simulink model "TrajectoryFollowVehicleWith14DoF_"  (R2024b)
settings: Solver=VariableStepAuto  StartTime=0  StopTime=14  FixedStep=timeStep  RelTol=1e-3
PreLoadFcn:
  | useDynamicsStanley = false; %Simulink model to move according to the scenario trajectory.
  | vehicleVariant = "3DOF";
PostLoadFcn:
  | load(fullfile(matlabroot,'toolbox','driving','drivingdata','rrScenarioSimTypes.mat'));
  | helperSLTrajectoryFollowerWithRRScenarioSetup();
  | hegihtMap = "flat";
  | if isfile("pathFollowingUtil/gridMap_groundHeight_RT.mat")
  |     load("gridMap_groundHeight_RT.mat");
  | end
  | % if exist("z_2DTable", "var") && exist("xBreakPts", "var") && exist("yBreakPts", "var")
  | %     hegihtMap = "2DMap";
  | % end
  | % if isfile("CRG/crgRoad.crg")
  | %     crgData = crg_read('CRG/crgRoad.crg');
  | % end
InitFcn:
  | if ~exist("slBus42", "var")
  |     load("Bus_VehFdbk.mat");
  | end
StartFcn:
  | % set_param(bdroot, 'Profile', 'on');
StopFcn:
  | % set_param(bdroot, 'Profile', 'off');
  | % slprofreport(bdroot, 'report14DoF.html');
undefined symbols (not defined in the file or in its folder): control_timeStep, Defined, Ego, egoInitialPose, egoInitialPoseCG, egoInitialPoseRear, InitVehicle, Lane, lr, m, magnitude, max_dc, n, Pose, RRtimeStep, SceneData, steerGear, tau, tau2, timeStep, User, VehicleData, Velocity, X, xBreakPts, Y, yBreakPts, Z, z_2DTable
libraries: sm_lib x40, nesl_utility x25, simulink_extras x12, sm_vehicle_utilities_lib x7, roadrunnerscenario x6, drivingvehiclecontroller x4, mpcadaslib x1, autolibshared x1
(part 1 of 3)
settings Model: Creator=The MathWorks, Inc.  LastModifiedBy=nobuakif
settings DataIOCC: SaveOutput=off  DSMLogging=off  InspectSignalLogs=on  SaveTime=off  ReturnWorkspaceOutputs=off
settings OptimizationCC: DefaultParameterBehavior=Inlined  ReuseModelBlockBuffer=off
settings DebuggingCC: ParameterTunabilityLossMsg=error  UnconnectedInputMsg=warning  UnconnectedOutputMsg=warning  UnconnectedLineMsg=warning
settings ModelReferenceCC: EnableRefExpFcnMdlSchedulingChecks=on  EnableParallelModelReferenceBuilds=on  PropagateSignalLabelsOutOfModel=off
settings RTWCC: GenCodeOnly=on  GenerateReport=on  GPUComputeCapability=3.5
settings CodeAppCC: ForceParamTrailComments=on
settings GRTTargetCC: TargetLangStandard=C89/C90 (ANSI)

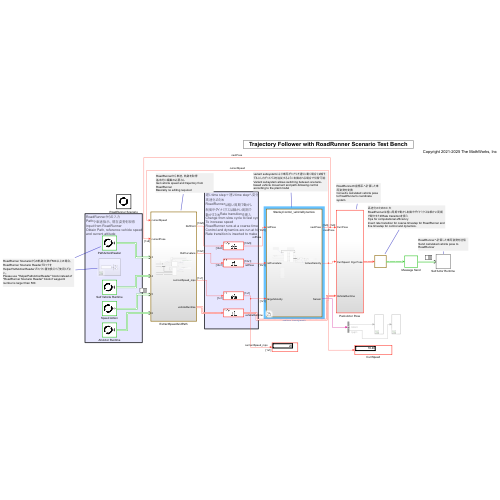
[thumbnail: Simulink's stored preview of the top-level diagram]
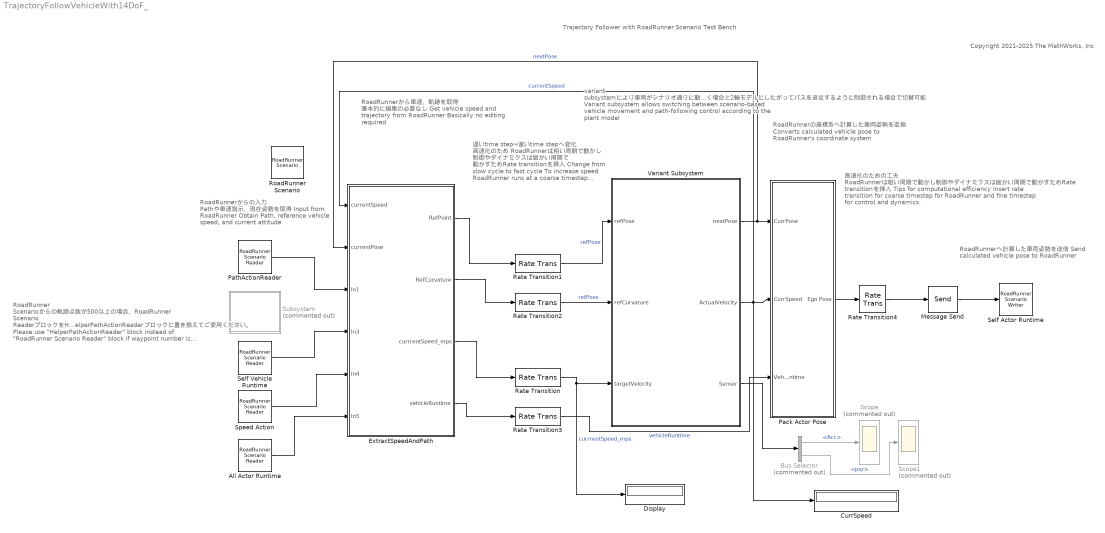
== system TrajectoryFollowVehicleWith14DoF_ ==
  note: 高速化のための工夫
      | RoadRunnerは粗い周期で動かし制御やダイナミクスは細かい周期で動かすためRate transitionを挿入
      | Tips for computational efficiency
      | Insert rate transition for coarse timestep for RoadRunner and fine timestep for control and dynamics.
  note: 遅いtime step⇒速いtime stepへ変化
      | 高速化のため
      | RoadRunnerは粗い周期で動かし
      | 制御やダイナミクスは細かい周期で
      | 動かすためRate transitionを挿入
      | Change from slow cycle to fast cycle
      | To increase speed
      | RoadRunner runs at a coarse timestep
      | Control and dynamics are run at high speed.
      | Rate transition is inserted to make control and dynamics run at high speed.
  note: RoadRunnerからの入力
      | Pathや車速指示、現在姿勢を取得
      | Input from RoadRunner
      | Obtain Path, reference vehicle speed,
      | and current attitude
  note: Trajectory Follower with RoadRunner Scenario Test Bench
  note: Copyright 2021-2025 The MathWorks, Inc
  note: RoadRunnerへ計算した車両姿勢を送信
      | Send calculated vehicle pose to RoadRunner
  note: RoadRunnerの座標系へ計算した車両姿勢を変換
      | Converts calculated vehicle pose to RoadRunner's coordinate system
  note: variant subsystemにより車両がシナリオ通りに動く場合と2輪モデルにしたがってパスを追従するように制御される場合で切替可能
      | Variant subsystem allows switching between scenario-based vehicle movement and path-following control according to the plant model
  note: RoadRunnerから車速、軌跡を取得
      | 基本的に編集の必要なし
      | Get vehicle speed and trajectory from RoadRunner
      | Basically no editing required
  note: RoadRunner Scenarioからの軌跡点数が500以上の場合、RoadRunner Scenario ReaderブロックをHelperPathActionReaderブロックに置き換えてご使用ください。
      | Please use "HelperPathActionReader" block instead of "RoadRunner Scenario Reader" block if waypoint number is larger than 500.
  All Actor Runtime : roadrunnerscenario/RoadRunner Scenario Reader  TopicCategory=Actor  ActorCategory=All Types  ActionType=Path Following  EventType=User-Defined  TopicType=Actor Pose  VehicleType=Vehicle Specifications  UserDefinedAction=Action1  UserDefinedEvent=Event1  Filter=None  SensorTopic=Target Poses  LaneBoundaryOutputTopic=Ego-Lane  SensorID=1  SampleTime=RRtimeStep
  Bus Selector : BusSelector  Commented=on  OutputSignals=IMU.Acc,IMU.pqr
  CurrSpeed : Display
  Display : Display
  ExtractSpeedAndPath : Subsystem
  Message Send : Send  OutputPortMessageModes=m
  Pack Actor Pose : Subsystem
  PathActionReader : roadrunnerscenario/RoadRunner Scenario Reader  TopicCategory=Action  ActorCategory=Vehicle  ActionType=Path Following  EventType=User-Defined  TopicType=Actor Specifications  VehicleType=Vehicle Pose  UserDefinedAction=Action1  UserDefinedEvent=Event1  Filter=Self  SensorTopic=Target Poses  LaneBoundaryOutputTopic=Ego-Lane  SensorID=1  SampleTime=RRtimeStep
  Rate Transition{,1..3} (4 alike) : RateTransition  OutPortSampleTime=timeStep
  Rate Transition4 : RateTransition  OutPortSampleTime=RRtimeStep
  RoadRunner Scenario : roadrunnerscenario/RoadRunner Scenario  UserDefinedActions={}  UserDefinedEvents={}
  Scope : Scope  Commented=on
  Scope1 : Scope  Commented=on
  Self Actor Runtime : roadrunnerscenario/RoadRunner Scenario Writer  TopicCategory=Actor  ActorCategory=All Types  EventType=Action Complete  UserDefinedEvent=Event1  VehicleType=Vehicle Pose  TopicType=Actor Pose
  Self Vehicle Runtime : roadrunnerscenario/RoadRunner Scenario Reader  TopicCategory=Actor  ActorCategory=Vehicle  ActionType=Path Following  EventType=User-Defined  TopicType=Actor Specifications  VehicleType=Vehicle Pose  UserDefinedAction=Action1  UserDefinedEvent=Event1  Filter=Self  SensorTopic=Target Poses  LaneBoundaryOutputTopic=Ego-Lane  SensorID=1  SampleTime=RRtimeStep
  Speed Action : roadrunnerscenario/RoadRunner Scenario Reader  TopicCategory=Action  ActorCategory=All Types  ActionType=Speed Change  EventType=User-Defined  TopicType=Actor Specifications  VehicleType=Vehicle Specifications  UserDefinedAction=Action1  UserDefinedEvent=Event1  Filter=Self  SensorTopic=Target Poses  LaneBoundaryOutputTopic=Ego-Lane  SensorID=1  SampleTime=RRtimeStep
  Subsystem : Subsystem  Commented=on
  Variant Subsystem : Subsystem  Variant=on
  wires:
  Rate Transition/1 -> Display/1, Variant Subsystem/3(targetVelocity)  "currrentSpeed_mps"
  ExtractSpeedAndPath/4(vehicleRuntime) -> Rate Transition3/1
  Pack Actor Pose/1(Ego Pose) -> Rate Transition4/1
  Message Send/1 -> Self Actor Runtime/1
  Rate Transition4/1 -> Message Send/1
  Rate Transition1/1 -> Variant Subsystem/1(refPose)  "refPose"
  Variant Subsystem/2(ActualVelocity) -> ExtractSpeedAndPath/1(currentSpeed), CurrSpeed/1, Pack Actor Pose/2(CurrSpeed)  "currentSpeed"
  Variant Subsystem/1(nextPose) -> ExtractSpeedAndPath/2(currentPose), Pack Actor Pose/1(CurrPose)  "nextPose"
  Rate Transition2/1 -> Variant Subsystem/2(refCurvature)  "refPose"
  PathActionReader/1 -> ExtractSpeedAndPath/3(In1)
  Self Vehicle Runtime/1 -> ExtractSpeedAndPath/4(In3)
  Speed Action/1 -> ExtractSpeedAndPath/5(In4)
  All Actor Runtime/1 -> ExtractSpeedAndPath/6(In5)
  ExtractSpeedAndPath/1(RefPoint) -> Rate Transition1/1
  ExtractSpeedAndPath/2(RefCurvature) -> Rate Transition2/1
  ExtractSpeedAndPath/3(currrentSpeed_mps) -> Rate Transition/1
  Rate Transition3/1 -> Pack Actor Pose/3(VehicleRuntime)  "vehicleRuntime"
  Variant Subsystem/3(Sensor) -> Bus Selector/1
  Bus Selector/1 -> Scope/1  "<Acc>"
  Bus Selector/2 -> Scope1/1  "<pqr>"

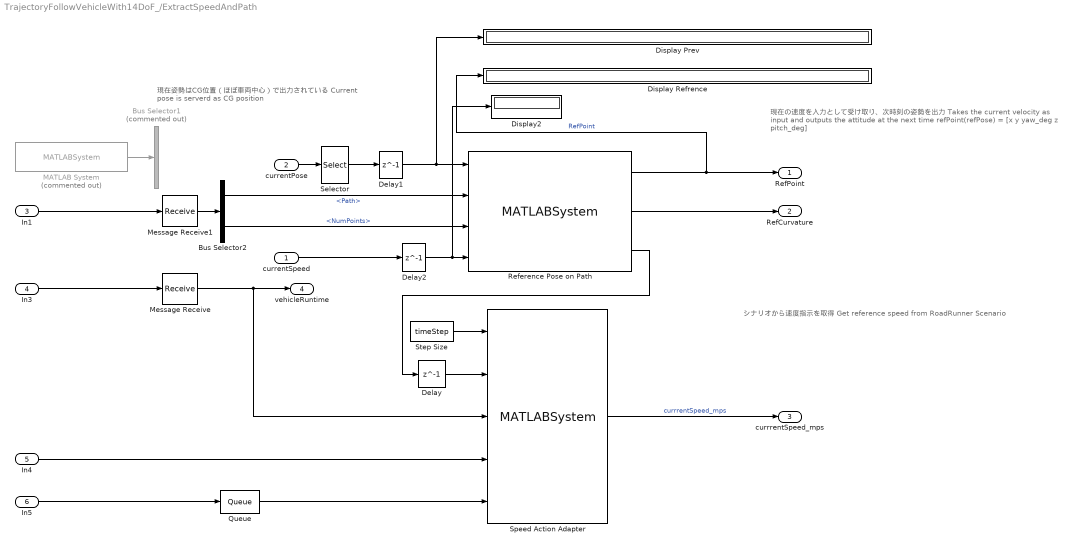
== system TrajectoryFollowVehicleWith14DoF_/ExtractSpeedAndPath ==
  note: 現在の速度を入力として受け取り、次時刻の姿勢を出力
      | Takes the current velocity as input and outputs the attitude at the next time
      | refPoint(refPose) = [x y yaw_deg z pitch_deg]
  note: シナリオから速度指示を取得
      | Get reference speed from RoadRunner Scenario
  note: 現在姿勢はCG位置（ほぼ車両中心）で出力されている
      | Current pose is serverd as CG position
  currentSpeed : Inport
  currentPose : Inport  Port=2
  In1 : Inport  Port=3
  In3 : Inport  Port=4
  In4 : Inport  Port=5
  In5 : Inport  Port=6
  Bus Selector1 : BusSelector  Commented=on  OutputSignals=Path,NumPoints
  Bus Selector2 : BusSelector  OutputSignals=PathTarget.Path,PathTarget.NumPoints
  Delay : Delay  DelayLength=1  InitialCondition=logical(0)
  Delay1 : Delay  DelayLength=1  InitialCondition=egoInitialPoseCG.CurrPose
  Delay2 : Delay  DelayLength=1  InitialCondition=norm(egoInitialPose.Velocity)
  Display Prev : Display
  Display Refrence : Display
  Display2 : Display
  MATLAB System : MATLABSystem  Commented=on  System=HelperPathActionReader  sampleTime=-1
      mask Type: HelperPathActionReader
      mask Display:
      | disp('HelperPathActionReader');
      | port_label('output',1,'PathTarget');
  Message Receive : Receive  InputPortMessageModes=m
  Message Receive1 : Receive  InputPortMessageModes=m
  Queue : Queue  InputPortMessageModes=m  OutputPortMessageModes=m  OverwriteOldest=on  Capacity=16  QueueType=LIFO
  Reference Pose on Path : MATLABSystem  System=HelperReferencePoseOnPath  timeStep=timeStep  vehicleOnPath=useDynamicsStanley == false  long_offset=refPts_offset  debugFig=false  saveFigVideo=false  zoomFig=nan  searchIndx=10  numReferencePose=numReferencePose  controlTimestep=0.1
      mask Type: HelperReferencePoseOnPath
      mask Display:
      | disp(['HelperReferencePoseOnPath' char(10) '' char(10) '' char(10) '' char(10) '']);
      | port_label('input',1,'PrevVehicleInfo');
      | port_label('input',2,'Trajectory');
      | port_label('input',3,'NumTrajPoints');
      | port_label('input',4,'currentSpeed');
      | port_label('output',1,'RefPointOnPath');
      | port_label('output',2,'RefCurvature');
      | port_label('output',3,'IsGoalReached');
  Selector : Selector  InputPortWidth=6  IndexOptions=Index vector (dialog)  Indices=1:5  OutputSizes=1
  Speed Action Adapter : MATLABSystem  InputPortMessageModes=n,n,n,m,m  System=HelperSpeedActionAdapter
      mask Type: HelperSpeedActionAdapter
      mask Display:
      | disp(['HelperSpeedActionAdapter' char(10) '' char(10) '']);
      | port_label('input',1,'timestep');
      | port_label('input',2,'stopVehicle');
      | port_label('input',3,'vehicleRuntime');
      | port_label('input',4,'msgSpeedAction');
      | port_label('input',5,'msgAllVehicleRuntime');
      | port_label('output',1,'currentSpeed');
  Step Size : Constant  Value=timeStep
  RefPoint : Outport
  RefCurvature : Outport  Port=2
  currrentSpeed_mps : Outport  Port=3
  vehicleRuntime : Outport  Port=4
  wires:
  Delay/1 -> Speed Action Adapter/2
  Reference Pose on Path/1 -> Display Refrence/1, RefPoint/1  "RefPoint"
  Step Size/1 -> Speed Action Adapter/1
  Message Receive1/1 -> Bus Selector2/1
  Reference Pose on Path/3 -> Delay/1
  Bus Selector2/1 -> Reference Pose on Path/2  "<Path>"
  Message Receive/1 -> vehicleRuntime/1, Speed Action Adapter/3
  In4/1 -> Speed Action Adapter/4
  Bus Selector2/2 -> Reference Pose on Path/3  "<NumPoints>"
  In3/1 -> Message Receive/1
  Reference Pose on Path/2 -> RefCurvature/1
  In5/1 -> Queue/1
  Speed Action Adapter/1 -> currrentSpeed_mps/1  "currrentSpeed_mps"
  In1/1 -> Message Receive1/1
  currentSpeed/1 -> Delay2/1
  Queue/1 -> Speed Action Adapter/5
  Delay1/1 -> Reference Pose on Path/1, Display Prev/1
  currentPose/1 -> Selector/1
  Selector/1 -> Delay1/1
  Delay2/1 -> Reference Pose on Path/4, Display2/1
  MATLAB System/1 -> Bus Selector1/1

== system TrajectoryFollowVehicleWith14DoF_/Pack Actor Pose ==
  CurrPose : Inport
  CurrSpeed : Inport  Port=2
  VehicleRuntime : Inport  Port=3
  Assign : BusAssignment  AssignedSignals=Pose,Velocity
  Bus Selector : BusSelector  OutputSignals=ActorRuntime
  Cvt2RRSCoodinate : MATLAB Function  TreatAsAtomicUnit=on
  Display : Display
  Pose Generation : MATLAB Function  TreatAsAtomicUnit=on
  Selector : Selector  InputPortWidth=6  IndexOptions=Index vector (dialog)  Indices=[3, 5]  OutputSizes=1
  Velocity XYZ Components : MATLAB Function  TreatAsAtomicUnit=on
  Ego Pose : Outport
  wires:
  Velocity XYZ Components/1(velocity) -> Display/1, Assign/3  "Velocity"
  Pose Generation/1(currPose) -> Assign/2  "Pose"
  Selector/1 -> Velocity XYZ Components/1(yaw_pitch)
  CurrSpeed/1 -> Velocity XYZ Components/2(speed)
  VehicleRuntime/1 -> Bus Selector/1
  Bus Selector/1 -> Assign/1  "<ActorRuntime>"
  Assign/1 -> Ego Pose/1
  CurrPose/1 -> Selector/1, Cvt2RRSCoodinate/1(pose)
  Cvt2RRSCoodinate/1(RRSPose) -> Pose Generation/1(pose)

== system TrajectoryFollowVehicleWith14DoF_/Subsystem ==
  Bus Selector2 : BusSelector  OutputSignals=PathTarget.Path,PathTarget.NumPoints
  MATLAB System : MATLABSystem  System=HelperPathActionReader  sampleTime=-1
      mask Type: HelperPathActionReader
      mask Display:
      | disp('HelperPathActionReader');
      | port_label('output',1,'PathTarget');
  Terminator1 : Terminator
  Terminator2 : Terminator
  wires:
  Bus Selector2/2 -> Terminator2/1  "<NumPoints>"
  MATLAB System/1 -> Bus Selector2/1
  Bus Selector2/1 -> Terminator1/1  "<Path>"

== system TrajectoryFollowVehicleWith14DoF_/Variant Subsystem ==
  refPose : Inport
  refCurvature : Inport  Port=2
  targetVelocity : Inport  Port=3
  IdealVehicleDynamics : Subsystem  VariantControl=useDynamicsStanley == false
  StanleyControl_vehicleDynamics : Subsystem  VariantControl=useDynamicsStanley == true
  nextPose : Outport
  ActualVelocity : Outport  Port=2
  Sensor : Outport  Port=3

== system TrajectoryFollowVehicleWith14DoF_/Variant Subsystem/IdealVehicleDynamics ==
  refPose : Inport
  refCurvature : Inport  Port=2
  targetVelocity : Inport  Port=3
  Terminator : Terminator
  Vector Concatenate : Concatenate
  Zero : Constant  Value=0  OutDataTypeStr=Inherit: Inherit via back propagation
  nextPose : Outport
  ActualVelocity : Outport  Port=2
  wires:
  targetVelocity/1 -> ActualVelocity/1
  refCurvature/1 -> Terminator/1
  refPose/1 -> Vector Concatenate/1
  Vector Concatenate/1 -> nextPose/1
  Zero/1 -> Vector Concatenate/2

== system TrajectoryFollowVehicleWith14DoF_/Variant Subsystem/StanleyControl_vehicleDynamics ==
  note: 車両ダイナミクスブロック
      | 2輪モデル、14自由度のフルビークルモデル、Simscape Multibodyでのフルビークルモデルを切り替えて使用可能
      | Vehicle Dynamics Block
      | Switch between bicycle models, full vehicle models with 14 degrees of freedom, and full vehicle models with Simscape Multibody
  note: 制御ブロック
      | 参照軌跡と参照車速に収束するようにステアリング角度、加速指示、減速指示を出力
      | Control block
      | Outputs steering angle, acceleration instructions, and deceleration instructions to converge with reference trajectory and reference vehicle speed
  note: bicycleモデルの場合、z値やピッチの情報がないためRoadRunner Sceanrioからの参照値を追加
      | For bicycle models, add reference values from RoadRunner Sceanrio as there is no z-value or pitch information
  refPose : Inport
  refCurvature : Inport  Port=2
  targetVelocity : Inport  Port=3
  Bus Selector : BusSelector  OutputSignals=CurrPose
  Bus Selector2 : BusSelector  Commented=on  OutputSignals=CurrPose
  Delay1 : Delay  DelayLength=1  InitialCondition=egoInitialPoseRear
  Lateral Metrics : MATLAB Function  Commented=on  TreatAsAtomicUnit=on
  Override Z and Pitch : Subsystem  Variant=on
  Stanley Controller : Subsystem  Commented=on
  Terminator : Terminator  Commented=on
  Terminator1 : Terminator  Commented=on
  Variant Subsystem : Subsystem  Variant=on
  Vehicle Dynamics1 : Subsystem  Variant=on  VariantControl=Vehicle Dynamics
  nextPose : Outport
  ActualVelocity : Outport  Port=2
  Sensor : Outport  Port=3
  wires:
  Vehicle Dynamics1/1(VehicleInfoRear) -> Delay1/1
  Vehicle Dynamics1/2(Speed) -> ActualVelocity/1  "speed"
  Bus Selector/1 -> Override Z and Pitch/1(currPose)  "<CurrPose>"
  Lateral Metrics/2(headingError) -> Terminator1/1  "relative_heading"
  Bus Selector2/1 -> Lateral Metrics/1(currPose)  "<CurrPose>"
  Lateral Metrics/1(positionError) -> Terminator/1  "position_error"
  Vehicle Dynamics1/4(Sensor) -> Sensor/1
  Override Z and Pitch/1(Out1) -> Bus Selector2/1, nextPose/1
  [refPose] -> Override Z and Pitch/2(refPose)
  Vehicle Dynamics1/3(VehicleInfoCG) -> Bus Selector/1
  Delay1/1 -> Variant Subsystem/1(VehicleInfo)
  refPose/1 -> Variant Subsystem/2(RefPose), [refPose]
  refCurvature/1 -> Variant Subsystem/3(Curvature)
  targetVelocity/1 -> Variant Subsystem/4(Speed)
  Variant Subsystem/1(SteerCmd) -> Vehicle Dynamics1/1(Steering Angle)
  Variant Subsystem/2(AccelCmd) -> Vehicle Dynamics1/2(Acceleration)
  Variant Subsystem/3(DecelCmd) -> Vehicle Dynamics1/3(Deceleration)

== system TrajectoryFollowVehicleWith14DoF_/Variant Subsystem/StanleyControl_vehicleDynamics/Override Z and Pitch ==
  note: 1) Add Subsystem or Model blocks as valid variant choices.
      | 2) You cannot connect blocks at this level. At simulation, connectivity is automatically
      | determined, based on the active variant and port name matching.
  currPose : Inport
  refPose : Inport  Port=2
  notOverride : Subsystem  VariantControl="vehicleVariant == \"14DOF\" || vehicleVariant == \"Multibody\""
  override : Subsystem  VariantControl="vehicleVariant == \"3DOF\""
  Out1 : Outport

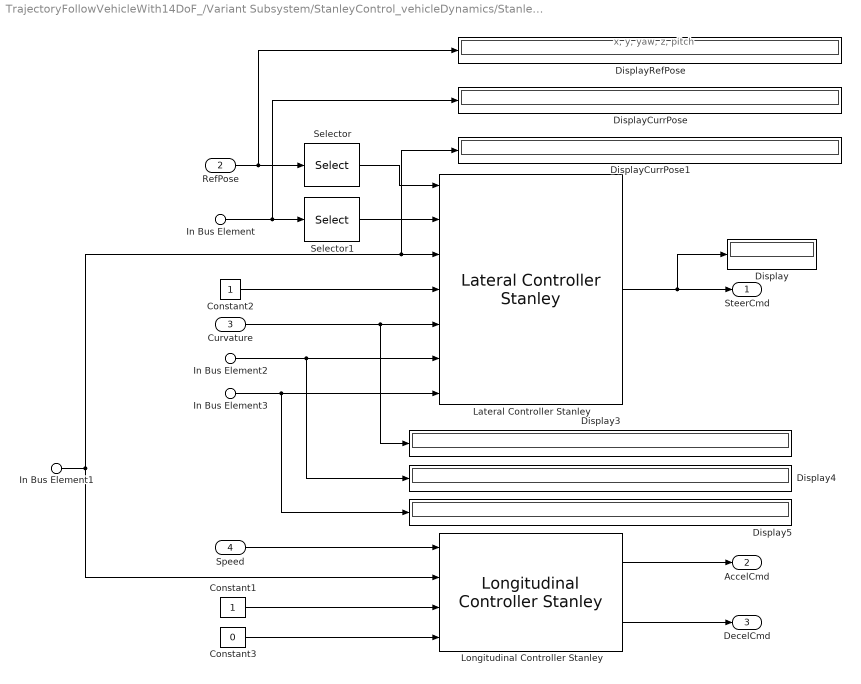
== system TrajectoryFollowVehicleWith14DoF_/Variant Subsystem/StanleyControl_vehicleDynamics/Stanley Controller ==
  note: x, y, yaw, z, pitch
  In Bus Element : Inport  PortName=VehicleInfo  Element=CurrPose
  In Bus Element1 : Inport  PortName=VehicleInfo  Element=CurrVelocity
  In Bus Element2 : Inport  PortName=VehicleInfo  Element=CurrYawRate
  In Bus Element3 : Inport  PortName=VehicleInfo  Element=CurrSteer
  RefPose : Inport  Port=2
  Curvature : Inport  Port=3
  Speed : Inport  Port=4
  Constant1 : Constant
  Constant2 : Constant
  Constant3 : Constant  Value=0
  Display{,3..5} (4 alike) : Display
  DisplayCurrPose : Display
  DisplayCurrPose1 : Display
  DisplayRefPose : Display
  Lateral Controller Stanley : drivingvehiclecontroller/Lateral Controller Stanley  ModelType=Dynamic bicycle model  PositionGainF=3  PositionGainR=2.5  YawRateGain=0.2  DelayGain=0.2  VehicleMass=m  Lf=lf  Lr=lr  TireStiffness=Cf  Wheelbase=2.8  MaxSteeringAngle=steerLimit
  Longitudinal Controller Stanley : drivingvehiclecontroller/Longitudinal Controller Stanley  Kp=2  Ki=1  SampleTime=timeStep  MaxAcceleration=max_ac  MaxDeceleration=max_dc
  Selector : Selector  InputPortWidth=5  IndexOptions=Index vector (dialog)  Indices=[1:3]  OutputSizes=1
  Selector1 : Selector  InputPortWidth=5  IndexOptions=Index vector (dialog)  Indices=[1:3]  OutputSizes=1
  SteerCmd : Outport
  AccelCmd : Outport  Port=2
  DecelCmd : Outport  Port=3
  wires:
  In Bus Element/1 -> DisplayCurrPose/1, Selector1/1
  Lateral Controller Stanley/1 -> Display/1, SteerCmd/1
  In Bus Element2/1 -> Display4/1, Lateral Controller Stanley/6
  In Bus Element1/1 -> DisplayCurrPose1/1, Lateral Controller Stanley/3, Longitudinal Controller Stanley/2
  Constant1/1 -> Longitudinal Controller Stanley/3
  Longitudinal Controller Stanley/2 -> DecelCmd/1
  Constant2/1 -> Lateral Controller Stanley/4
  In Bus Element3/1 -> Display5/1, Lateral Controller Stanley/7
  Constant3/1 -> Longitudinal Controller Stanley/4
  RefPose/1 -> DisplayRefPose/1, Selector/1
  Longitudinal Controller Stanley/1 -> AccelCmd/1
  Curvature/1 -> Display3/1, Lateral Controller Stanley/5
  Speed/1 -> Longitudinal Controller Stanley/1
  Selector/1 -> Lateral Controller Stanley/1
  Selector1/1 -> Lateral Controller Stanley/2

== system TrajectoryFollowVehicleWith14DoF_/Variant Subsystem/StanleyControl_vehicleDynamics/Variant Subsystem ==
  note: 1) Add Subsystem or Model blocks as valid variant choices.
      | 2) You cannot connect blocks at this level. At simulation, connectivity is automatically
      | determined, based on the active variant and port name matching.
  VehicleInfo : Inport
  RefPose : Inport  Port=2
  Curvature : Inport  Port=3
  Speed : Inport  Port=4
  MPC : Subsystem  VariantControl="controlMode == \"mpc\""
  Stanley : Subsystem  VariantControl="controlMode == \"stanley\""
  mpc_mod : ModelReference  ModelNameDialog=mpc_pathFollowingMod.slx  SimulationMode=Normal  VariantControl="controlMode == \"mpc_mod\""  ModelReferenceVersion=1.86
  SteerCmd : Outport
  AccelCmd : Outport  Port=2
  DecelCmd : Outport  Port=3

== system TrajectoryFollowVehicleWith14DoF_/Variant Subsystem/StanleyControl_vehicleDynamics/Vehicle Dynamics1 ==
  Steering Angle : Inport
  Acceleration : Inport  Port=2
  Deceleration : Inport  Port=3
  Vehicle Dynamics 14DOF : Subsystem  VariantControl="vehicleVariant == \"14DOF\""
  Vehicle Dynamics 3DOF : Subsystem  VariantControl="vehicleVariant == \"3DOF\""
  Vehicle Dynamics Multibody : Subsystem  VariantControl="vehicleVariant == \"Multibody\""
  VehicleInfoRear : Outport
  Speed : Outport  Port=2
  VehicleInfoCG : Outport  Port=3
  Sensor : Outport  Port=4

== system TrajectoryFollowVehicleWith14DoF_/Variant Subsystem/StanleyControl_vehicleDynamics/Override Z and Pitch/notOverride ==
  currPose : Inport
  Out1 : Outport
  wires:
  currPose/1 -> Out1/1

== system TrajectoryFollowVehicleWith14DoF_/Variant Subsystem/StanleyControl_vehicleDynamics/Override Z and Pitch/override ==
  currPose : Inport
  refPose : Inport  Port=2
  Constant : Constant  Value=0
  Mux : Mux  Inputs=3
  Selector : Selector  InputPortWidth=5  IndexOptions=Index vector (dialog)  Indices=[4:5]  OutputSizes=1
  Selector1 : Selector  InputPortWidth=6  IndexOptions=Index vector (dialog)  Indices=1:3  OutputSizes=1
  Selector2 : Selector  NumberOfDimensions=2  InputPortWidth=30  IndexOptions=Index vector (dialog),Select all  Indices=1,1  OutputSizes=1,1
  Out1 : Outport
  wires:
  Mux/1 -> Out1/1
  refPose/1 -> Selector2/1
  currPose/1 -> Selector1/1
  Selector1/1 -> Mux/1
  Selector/1 -> Mux/2
  Constant/1 -> Mux/3
  Selector2/1 -> Selector/1

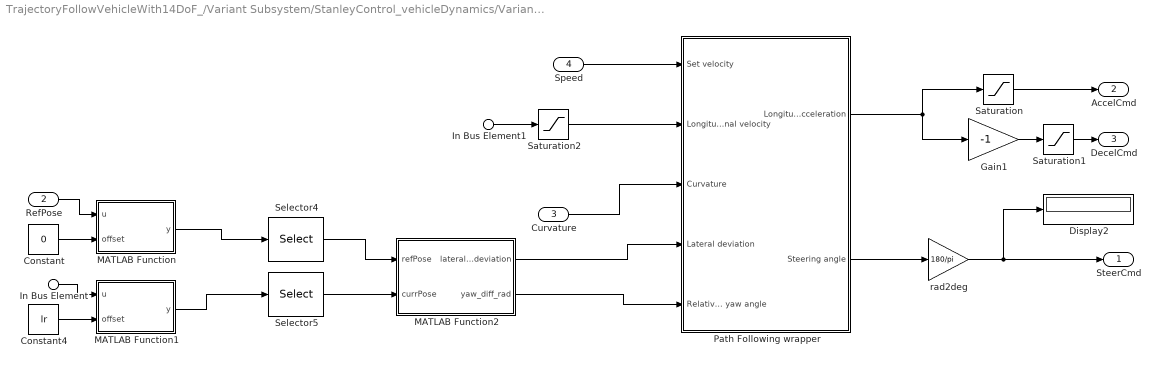
== system TrajectoryFollowVehicleWith14DoF_/Variant Subsystem/StanleyControl_vehicleDynamics/Variant Subsystem/MPC ==
  In Bus Element : Inport  PortName=VehicleInfo  Element=CurrPose
  In Bus Element1 : Inport  PortName=VehicleInfo  Element=CurrVelocity
  RefPose : Inport  Port=2
  Curvature : Inport  Port=3
  Speed : Inport  Port=4
  Constant : Constant  Value=0
  Constant4 : Constant  Value=lr
  Display2 : Display
  Gain1 : Gain  Gain=-1
  MATLAB Function : MATLAB Function  TreatAsAtomicUnit=on
  MATLAB Function1 : MATLAB Function  TreatAsAtomicUnit=on
  MATLAB Function2 : MATLAB Function  TreatAsAtomicUnit=on
  Path Following wrapper : Subsystem  Variant=on
  Saturation : Saturate  UpperLimit=inf  LowerLimit=0
  Saturation1 : Saturate  UpperLimit=inf  LowerLimit=0
  Saturation2 : Saturate  UpperLimit=inf  LowerLimit=0.01
  Selector4 : Selector  InputPortWidth=5  IndexOptions=Index vector (dialog)  Indices=[1:3]  OutputSizes=1
  Selector5 : Selector  InputPortWidth=5  IndexOptions=Index vector (dialog)  Indices=[1:3]  OutputSizes=1
  rad2deg : Gain  Gain=180/pi
  SteerCmd : Outport
  AccelCmd : Outport  Port=2
  DecelCmd : Outport  Port=3
  wires:
  RefPose/1 -> MATLAB Function/1(u)
  In Bus Element/1 -> MATLAB Function1/1(u)
  Constant/1 -> MATLAB Function/2(offset)
  Constant4/1 -> MATLAB Function1/2(offset)
  MATLAB Function/1(y) -> Selector4/1
  MATLAB Function1/1(y) -> Selector5/1
  Path Following wrapper/1(Longitudinal acceleration) -> Gain1/1, Saturation/1
  MATLAB Function2/2(yaw_diff_rad) -> Path Following wrapper/5(Relative yaw angle)
  Selector4/1 -> MATLAB Function2/1(refPose)
  Selector5/1 -> MATLAB Function2/2(currPose)
  Speed/1 -> Path Following wrapper/1(Set velocity)
  In Bus Element1/1 -> Saturation2/1
  MATLAB Function2/1(lateral_deviation) -> Path Following wrapper/4(Lateral deviation)
  Path Following wrapper/2(Steering angle) -> rad2deg/1
  Saturation/1 -> AccelCmd/1
  Saturation1/1 -> DecelCmd/1
  rad2deg/1 -> SteerCmd/1, Display2/1
  Saturation2/1 -> Path Following wrapper/2(Longitudinal velocity)
  Gain1/1 -> Saturation1/1
  Curvature/1 -> Path Following wrapper/3(Curvature)

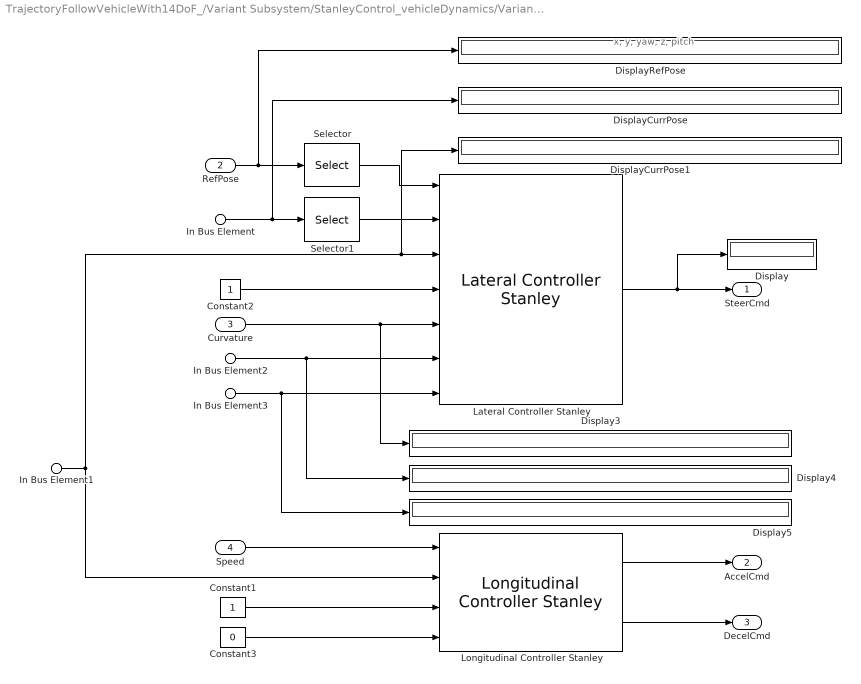
== system TrajectoryFollowVehicleWith14DoF_/Variant Subsystem/StanleyControl_vehicleDynamics/Variant Subsystem/Stanley ==
  note: x, y, yaw, z, pitch
  In Bus Element : Inport  PortName=VehicleInfo  Element=CurrPose
  In Bus Element1 : Inport  PortName=VehicleInfo  Element=CurrVelocity
  In Bus Element2 : Inport  PortName=VehicleInfo  Element=CurrYawRate
  In Bus Element3 : Inport  PortName=VehicleInfo  Element=CurrSteer
  RefPose : Inport  Port=2
  Curvature : Inport  Port=3
  Speed : Inport  Port=4
  Constant1 : Constant
  Constant2 : Constant
  Constant3 : Constant  Value=0
  Display{,3..5} (4 alike) : Display
  DisplayCurrPose : Display
  DisplayCurrPose1 : Display
  DisplayRefPose : Display
  Lateral Controller Stanley : drivingvehiclecontroller/Lateral Controller Stanley  ModelType=Dynamic bicycle model  PositionGainF=3  PositionGainR=2.5  YawRateGain=0.2  DelayGain=0.2  VehicleMass=m  Lf=lf  Lr=lr  TireStiffness=Cf  Wheelbase=2.8  MaxSteeringAngle=steerLimit
  Longitudinal Controller Stanley : drivingvehiclecontroller/Longitudinal Controller Stanley  Kp=2  Ki=1  SampleTime=timeStep  MaxAcceleration=max_ac  MaxDeceleration=max_dc
  Selector : Selector  InputPortWidth=5  IndexOptions=Index vector (dialog)  Indices=[1:3]  OutputSizes=1
  Selector1 : Selector  InputPortWidth=5  IndexOptions=Index vector (dialog)  Indices=[1:3]  OutputSizes=1
  SteerCmd : Outport
  AccelCmd : Outport  Port=2
  DecelCmd : Outport  Port=3
  wires:
  In Bus Element/1 -> DisplayCurrPose/1, Selector1/1
  In Bus Element3/1 -> Display5/1, Lateral Controller Stanley/7
  In Bus Element2/1 -> Display4/1, Lateral Controller Stanley/6
  In Bus Element1/1 -> DisplayCurrPose1/1, Lateral Controller Stanley/3, Longitudinal Controller Stanley/2
  Constant2/1 -> Lateral Controller Stanley/4
  Selector/1 -> Lateral Controller Stanley/1
  Constant1/1 -> Longitudinal Controller Stanley/3
  Speed/1 -> Longitudinal Controller Stanley/1
  Selector1/1 -> Lateral Controller Stanley/2
  Curvature/1 -> Display3/1, Lateral Controller Stanley/5
  Lateral Controller Stanley/1 -> Display/1, SteerCmd/1
  Longitudinal Controller Stanley/2 -> DecelCmd/1
  Longitudinal Controller Stanley/1 -> AccelCmd/1
  RefPose/1 -> DisplayRefPose/1, Selector/1
  Constant3/1 -> Longitudinal Controller Stanley/4

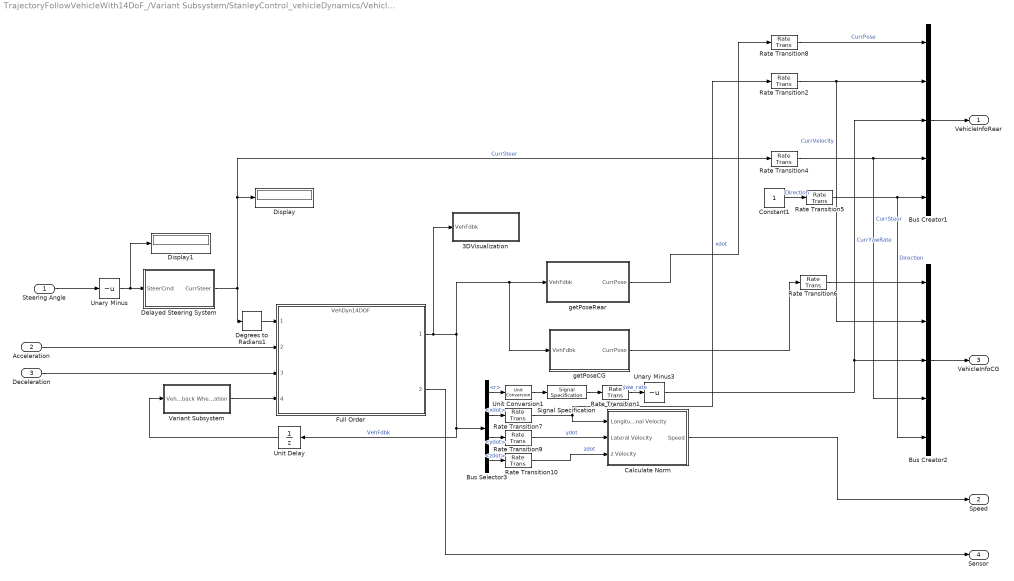
== system TrajectoryFollowVehicleWith14DoF_/Variant Subsystem/StanleyControl_vehicleDynamics/Vehicle Dynamics1/Vehicle Dynamics 14DOF ==
  Steering Angle : Inport
  Acceleration : Inport  Port=2
  Deceleration : Inport  Port=3
  3DVisualization : Subsystem  Variant=on
  Bus Creator1 : BusCreator  Inputs=5  OutDataTypeStr=Bus: BusVehicleInfo  NonVirtualBus=on
      settings: InheritFromInputs=off
  Bus Creator2 : BusCreator  Inputs=5  OutDataTypeStr=Bus: BusFullVehicleInfo  NonVirtualBus=on
      settings: InheritFromInputs=off
  Bus Selector3 : BusSelector  OutputSignals=Body.BdyFrm.Cg.AngVel.r,Body.BdyFrm.Cg.Vel.xdot,Body.BdyFrm.Cg.Vel.ydot,Body.BdyFrm.Cg.Vel.zdot
  Calculate Norm : Subsystem
  Constant1 : Constant
  Degrees to Radians1 : simulink_extras/Transformations/Degrees to Radians
  Delayed Steering System : Subsystem
  Display : Display
  Display1 : Display
  Full Order : ModelReference  ModelNameDialog=VehDyn14DOF.slx  ModelReferenceVersion=8.48
  Rate Transition{1..2,4..10} (9 alike) : RateTransition  OutPortSampleTime=timeStep
  Signal Specification : SignalSpecification  Unit=deg/s
  Unary Minus : UnaryMinus
  Unary Minus3 : UnaryMinus
  Unit Conversion1 : UnitConversion
  Unit Delay : UnitDelay  SampleTime=-1  HasFrameUpgradeWarning=on
  Variant Subsystem : Subsystem  Variant=on
  getPoseCG : Subsystem
  getPoseRear : Subsystem
  VehicleInfoRear : Outport  VectorParamsAs1DForOutWhenUnconnected=off
  Speed : Outport  Port=2
  VehicleInfoCG : Outport  Port=3  VectorParamsAs1DForOutWhenUnconnected=off
  Sensor : Outport  Port=4  VectorParamsAs1DForOutWhenUnconnected=off
  wires:
  Calculate Norm/1(Speed) -> Speed/1
  Acceleration/1 -> Full Order/2
  Deceleration/1 -> Full Order/3
  Unary Minus/1 -> Display1/1, Delayed Steering System/1(SteerCmd)
  Degrees to Radians1/1 -> Full Order/1
  Full Order/1 -> Unit Delay/1, Bus Selector3/1, getPoseCG/1(VehFdbk), getPoseRear/1(VehFdbk), 3DVisualization/1(VehFdbk)  "VehFdbk"
  Variant Subsystem/1(WheelElevation) -> Full Order/4
  Rate Transition9/1 -> Calculate Norm/2(Lateral Velocity)  "ydot"
  Steering Angle/1 -> Unary Minus/1
  Rate Transition1/1 -> Unary Minus3/1  "yaw_rate"
  Delayed Steering System/1(CurrSteer) -> Display/1, Rate Transition4/1, Degrees to Radians1/1  "CurrSteer"
  Unary Minus3/1 -> Bus Creator1/3, Bus Creator2/3  "CurrYawRate"
  Rate Transition5/1 -> Bus Creator2/5, Bus Creator1/5  "Direction"
  Constant1/1 -> Rate Transition5/1  "Direction"
  Rate Transition6/1 -> Bus Creator2/1
  Rate Transition8/1 -> Bus Creator1/1  "CurrPose"
  Bus Creator2/1 -> VehicleInfoCG/1
  Bus Creator1/1 -> VehicleInfoRear/1
  Rate Transition2/1 -> Bus Creator2/2, Bus Creator1/2  "CurrVelocity"
  Rate Transition7/1 -> Calculate Norm/1(Longitudinal Velocity), Rate Transition2/1  "xdot"
  Rate Transition4/1 -> Bus Creator2/4, Bus Creator1/4  "CurrSteer"
  Full Order/2 -> Sensor/1
  Unit Delay/1 -> Variant Subsystem/1(VehFdback)
  Rate Transition10/1 -> Calculate Norm/3(z Velocity)  "zdot"
  Bus Selector3/4 -> Rate Transition10/1  "<zdot>"
  Bus Selector3/3 -> Rate Transition9/1  "<ydot>"
  Unit Conversion1/1 -> Signal Specification/1
  Bus Selector3/2 -> Rate Transition7/1  "<xdot>"
  Bus Selector3/1 -> Unit Conversion1/1  "<r>"
  Signal Specification/1 -> Rate Transition1/1
  getPoseRear/1(CurrPose) -> Rate Transition8/1
  getPoseCG/1(CurrPose) -> Rate Transition6/1

== system TrajectoryFollowVehicleWith14DoF_/Variant Subsystem/StanleyControl_vehicleDynamics/Vehicle Dynamics1/Vehicle Dynamics 3DOF ==
  Steering Angle : Inport
  Acceleration : Inport  Port=2
  Deceleration : Inport  Port=3
  Calculate Norm : Subsystem
  Data Type Conversion : DataTypeConversion  OutDataTypeStr=double  SaturateOnIntegerOverflow=off  RndMeth=Floor
  Degrees to Radians1 : simulink_extras/Transformations/Degrees to Radians
  Delayed Steering System : Subsystem
  Direction : Constant
  From : From
  Goto : Goto
  Pack Current States : Subsystem
  Rate Transition : RateTransition
  Simple Driveline & Brakes : Subsystem
  Terminator : Terminator
  Terminator1 : Terminator
  Terminator2 : Terminator
  Vehicle Body 3DOF Single Track : autolibshared/Vehicle Body 3DOF Single Track  trackMode=Single (bicycle)  inputMode=External longitudinal forces  frontSteerMode=on  rearSteerMode=off  windMode=off  muMode=off  extFMode=off  extMMode=off  htchFMode=off  htchMMode=off  extXo=off  extpsio=off  extxdoto=off  extro=off  extYo=off  extTamb=off  extydoto=off  aMode=2  NF=2  NR=2  m=m  a=lf  b=lr  h=0.35  dh=1  hh=0.2  X_o=egoInitialPoseCG.CurrPose(1)  xdot_o=egoInitialPoseCG.CurrVelocity  CalphaMode=off  sigmaMode=off  d=0  hl=0  w=[1.4,1.4]  Cy_f=Cf  Cy_r=Cr  sigma_f=.1  sigma_r=.1  alpha_f_brk=[-.1 .1]  Cy_f_data=[-9e3 9e3]  alpha_r_brk=[-.1 .1]  Cy_r_data=[-9e3 9e3]  Y_o=egoInitialPoseCG.CurrPose(2)  ydot_o=0  Izz=Iz  psi_o=deg2rad(egoInitialPoseCG.CurrPose(3))  r_o=deg2rad(egoInitialPoseCG.CurrYawRate)  Af=0  Cd=.3  Cl=.1  Cpm=.1  beta_w=[0:0.01:0.3]  Cs=[0:0.03:0.9]  Cym=[0:0.01:0.3]  Pabs=101325  Tair=273  g=9.81  mu=1  xdot_tol=.01  Fznom=5000  Fxtire_sat=7e4  Fytire_sat=7e4  longOff=0  latOff=0  vertOff=0  wrapAng=off
  VehicleInfoRear : Outport
  Speed : Outport  Port=2
  VehicleInfoCG : Outport  Port=3
  wires:
  Steering Angle/1 -> Delayed Steering System/1(SteerCmd)
  Acceleration/1 -> Simple Driveline & Brakes/1(Accel)
  Calculate Norm/1(Speed) -> Rate Transition/1
  Direction/1 -> Pack Current States/5(Direction), Simple Driveline & Brakes/3(Gear)
  Simple Driveline & Brakes/1(Front Force) -> Vehicle Body 3DOF Single Track/2
  Vehicle Body 3DOF Single Track/5 -> Pack Current States/4(CurrYawRate)
  Vehicle Body 3DOF Single Track/4 -> Terminator1/1
  Degrees to Radians1/1 -> Vehicle Body 3DOF Single Track/1
  Delayed Steering System/1(CurrSteer) -> Degrees to Radians1/1, Pack Current States/1(CurrSteer)
  Pack Current States/1(CurrVehicleInfoForDS) -> VehicleInfoRear/1
  Rate Transition/1 -> Speed/1
  Simple Driveline & Brakes/2(Rear Force) -> Vehicle Body 3DOF Single Track/3
  From/1 -> Calculate Norm/1(Lateral Velocity)
  Vehicle Body 3DOF Single Track/2 -> Data Type Conversion/1, Pack Current States/3(CurrVelocity)
  Vehicle Body 3DOF Single Track/6 -> Terminator/1
  Deceleration/1 -> Simple Driveline & Brakes/2(Decel)
  Vehicle Body 3DOF Single Track/7 -> Terminator2/1
  Vehicle Body 3DOF Single Track/3 -> Goto/1
  Data Type Conversion/1 -> Calculate Norm/2(Longitudinal Velocity), Simple Driveline & Brakes/4(xdot)
  Vehicle Body 3DOF Single Track/1 -> Pack Current States/2(Info)  "VehFdbk"
  Pack Current States/2(CurrVehicleInfoForRR) -> VehicleInfoCG/1

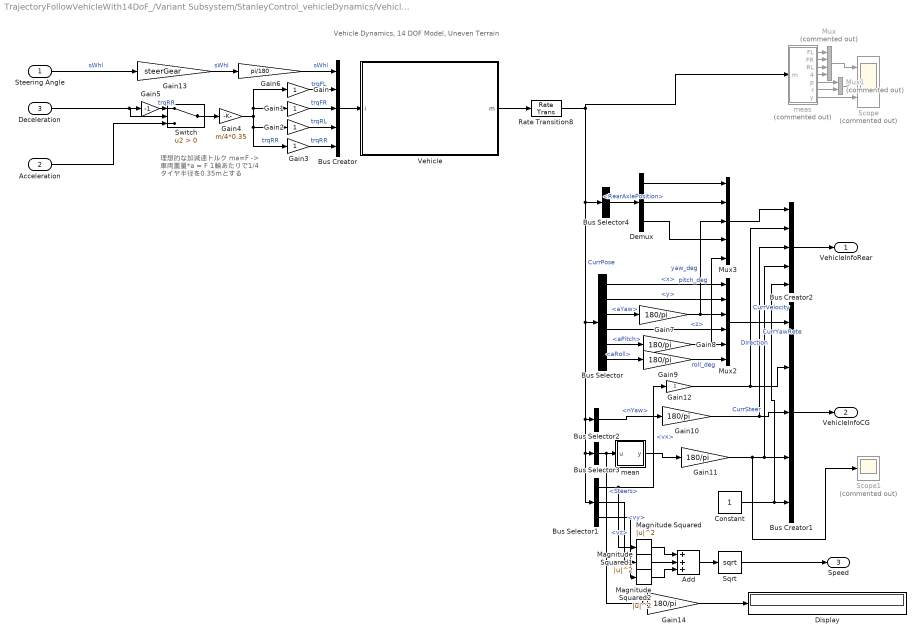
== system TrajectoryFollowVehicleWith14DoF_/Variant Subsystem/StanleyControl_vehicleDynamics/Vehicle Dynamics1/Vehicle Dynamics Multibody ==
  note: 理想的な加減速トルク
      | ma=F -> 車両重量*a = F
      | 1輪あたりで1/4
      | タイヤ半径を0.35mとする
  note: Vehicle Dynamics, 14 DOF Model, Uneven Terrain
  Steering Angle : Inport
  Acceleration : Inport  Port=2
  Deceleration : Inport  Port=3
  Add : Sum  Inputs=+++
  Bus Creator : BusCreator  Inputs=5
  Bus Creator1 : BusCreator  Inputs=5  OutDataTypeStr=Bus: BusFullVehicleInfo  NonVirtualBus=on
      settings: InheritFromInputs=off
  Bus Creator2 : BusCreator  Inputs=5  OutDataTypeStr=Bus: BusVehicleInfo  NonVirtualBus=on
      settings: InheritFromInputs=off
  Bus Selector : BusSelector  OutputSignals=Body.x,Body.y,Body.aYaw,Body.z,Body.aPitch,Body.aRoll
  Bus Selector1 : BusSelector  OutputSignals=Body.vx,Body.vy,Body.vz
  Bus Selector2 : BusSelector  OutputSignals=Body.nYaw
  Bus Selector3 : BusSelector  OutputSignals=Steers
  Bus Selector4 : BusSelector  OutputSignals=RearAxlePosition
  Constant : Constant
  Demux : Demux  Outputs=3
  Display : Display
  Gain{,1..3,12} (5 alike) : Gain
  Gain{7..11,14} (6 alike) : Gain  Gain=180/pi
  Gain13 : Gain  Gain=steerGear
  Gain4 : Gain  Gain=m/4*0.35
  Gain5 : Gain  Gain=-1
  Gain6 : Gain  Gain=pi/180
  Magnitude Squared : Math  Operator=magnitude^2
  Magnitude Squared1 : Math  Operator=magnitude^2
  Magnitude Squared2 : Math  Operator=magnitude^2
  Mux : Mux  Commented=on
  Mux1 : Mux  Commented=on  Inputs=2
  Mux2 : Mux  Inputs=6
  Mux3 : Mux  Inputs=5
  Rate Transition8 : RateTransition  OutPortSampleTime=timeStep
  Scope : Scope  Commented=on  NumInputPorts=3
  Scope1 : Scope  Commented=on
  Sqrt : Sqrt  OutputSignalType=real
  Switch : Switch  Criteria=u2 > Threshold  SaturateOnIntegerOverflow=off  InputSameDT=off
  Vehicle : Subsystem  mask(Vehicle and Scene){vehdata=VehicleData, initveh=InitVehicle}
      mask prompts: vehdata "Vehicle Data (structure)"; initveh "Initial Position, Velocity (structure)"
      mask help: Models a vehicle with a configurable scene. Vehicle parameters are defined within a single data structure. A separate data structure defines the initial position, orientation, and speed of the vehicle and the wheels.
      settings: AttributesFormatString=%<popup_scene>
      mask Display:
      | image(['sm_vehicle_2axle_heave_roll_vehicle_grid_ray_trace.png']);
      | % Notes for mask images
      | % Screenshot taken MechExp 931x463, one pane 619x314
      | % Trim to 434 x 272, resize to 500x330
  mean : MATLAB Function  TreatAsAtomicUnit=on
  meas : Subsystem  Commented=on
  VehicleInfoRear : Outport
  VehicleInfoCG : Outport  Port=2
  Speed : Outport  Port=3
  wires:
  Demux/3 -> Mux3/4
  Magnitude Squared2/1 -> Add/3
  Gain11/1 -> Scope1/1, Bus Creator1/4, Bus Creator2/4  "CurrSteer"
  Demux/1 -> Mux3/1
  Bus Creator1/1 -> VehicleInfoCG/1
  Bus Selector1/1 -> Gain12/1, Magnitude Squared/1  "<vx>"
  Bus Creator2/1 -> VehicleInfoRear/1
  Mux2/1 -> Bus Creator1/1
  Bus Selector/4 -> Mux2/4  "<z>"
  Gain13/1 -> Gain6/1  "sWhl"
  Gain6/1 -> Bus Creator/1  "sWhl"
  Sqrt/1 -> Speed/1
  Bus Selector1/2 -> Magnitude Squared1/1  "<vy>"
  Bus Selector3/1 -> Gain14/1, mean/1(u)  "<Steers>"
  Bus Selector/5 -> Gain8/1  "<aPitch>"
  Gain12/1 -> Bus Creator1/2, Bus Creator2/2  "CurrVelocity"
  Bus Selector2/1 -> Gain10/1  "<nYaw>"
  Gain10/1 -> Bus Creator2/3, Bus Creator1/3  "CurrYawRete"
  Bus Selector/1 -> Mux2/1  "<x>"
  Constant/1 -> Bus Creator2/5, Bus Creator1/5  "Direction"
  Mux3/1 -> Bus Creator2/1
  Bus Selector/2 -> Mux2/2  "<y>"
  Magnitude Squared/1 -> Add/1
  Magnitude Squared1/1 -> Add/2
  Gain7/1 -> Mux3/3, Mux2/3  "yaw_deg"
  Acceleration/1 -> Switch/3
  Mux/1 -> Scope/1
  meas/3(RL) -> Mux/3
  Demux/2 -> Mux3/2
  Bus Selector1/3 -> Magnitude Squared2/1  "<vz>"
  Vehicle/1(m) -> Rate Transition8/1
  Gain3/1 -> Bus Creator/5  "trqRR"
  Bus Selector/3 -> Gain7/1  "<aYaw>"
  Switch/1 -> Gain4/1
  Gain4/1 -> Gain1/1, Gain/1, Gain2/1, Gain3/1  "trqRR"
  Add/1 -> Sqrt/1
  Gain5/1 -> Switch/1  "trqRR"
  Gain/1 -> Bus Creator/2  "trqFL"
  mean/1(y) -> Gain11/1
  Bus Creator/1 -> Vehicle/1(i)
  meas/2(FR) -> Mux/2
  meas/1(FL) -> Mux/1
  Gain1/1 -> Bus Creator/3  "trqFR"
  Gain9/1 -> Mux2/6  "roll_deg"
  meas/6(r) -> Mux1/2
  meas/7(y) -> Scope/3
  Steering Angle/1 -> Gain13/1  "sWhl"
  Deceleration/1 -> Switch/2, Gain5/1
  Mux1/1 -> Scope/2
  meas/4(RR) -> Mux/4
  Gain8/1 -> Mux3/5, Mux2/5  "pitch_deg"
  Bus Selector4/1 -> Demux/1  "<RearAxlePosition>"
  Gain2/1 -> Bus Creator/4  "trqRL"
  Bus Selector/6 -> Gain9/1  "<aRoll>"
  meas/5(p) -> Mux1/1
  Rate Transition8/1 -> meas/1(m), Bus Selector1/1, Bus Selector3/1, Bus Selector2/1, Bus Selector/1, Bus Selector4/1  "CurrPose"
  Gain14/1 -> Display/1

== system TrajectoryFollowVehicleWith14DoF_/Variant Subsystem/StanleyControl_vehicleDynamics/Variant Subsystem/MPC/Path Following wrapper ==
  Set velocity : Inport
  Longitudinal velocity : Inport  Port=2
  Curvature : Inport  Port=3
  Lateral deviation : Inport  Port=4
  Relative yaw angle : Inport  Port=5
  Path Following Control System : mpcadaslib/Path Following Control System  VariantControl=true  ModelType=Use vehicle parameters  VehicleMass=m  VehicleYawInertia=Iz  LengthToFront=lf  LengthToRear=lr  FrontTireStiffness=Cf  RearTireStiffness=Cr  AccelTimeConstant=tau  EgoModelMatrixA=[-2,zeros(1,3);1,zeros(1,3);zeros(1,2),-4.4021,-12.4603;zeros(1,2),1.3913,-5.1868]  EgoModelMatrixB=[2,zeros(1,3);zeros(1,2),24.1270,15.8609]'  EgoModelMatrixC=[zeros(3,1),eye(3)]  InitialLongVel=norm(egoInitialPose.Velocity)  TransportLag=tau2  spaceCtrl=off  DefaultSpacing=0  MinSteering=min_steer  umin_ext=off  MaxSteering=max_steer  umax_ext=off  MinAcceleration=-max_dc  amin_ext=off  MaxAcceleration=max_ac  amax_ext=off  Ts=control_timeStep  PredictionHorizon=PredictionHorizon  ControlHorizon=3  LongWeight=0.1  LateralWeight=1  AccelRateWeight=0.1  SteerRateWeight=0.1  suboptimal=off  maxiter=10  datatypeopt=double  optmode=off  trackmode=off
      settings: LibrarySourceBlock=mpclib/Automated Driving/Path Following Control System
  Longitudinal acceleration : Outport  PortDimensions=1  VectorParamsAs1DForOutWhenUnconnected=off
  Steering angle : Outport  Port=2  VectorParamsAs1DForOutWhenUnconnected=off

== system TrajectoryFollowVehicleWith14DoF_/Variant Subsystem/StanleyControl_vehicleDynamics/Vehicle Dynamics1/Vehicle Dynamics 14DOF/3DVisualization ==
  note: 1) Add Subsystem or Model blocks as valid variant choices.
      | 2) You cannot connect blocks at this level. At simulation, connectivity is automatically
      | determined, based on the active variant and port name matching.
  VehFdbk : Inport
  3D Engine : ModelReference  ModelNameDialog=sim3d_visualization.slx  SimulationMode=Normal  VariantControl=debug_engine3D==true  ModelReferenceVersion=5.2
  No 3D Engine : Subsystem  VariantControl=debug_engine3D==false

== system TrajectoryFollowVehicleWith14DoF_/Variant Subsystem/StanleyControl_vehicleDynamics/Vehicle Dynamics1/Vehicle Dynamics 14DOF/Calculate Norm ==
  Longitudinal Velocity : Inport
  Lateral Velocity : Inport  Port=2
  z Velocity : Inport  Port=3
  Add : Sum  Inputs=+++
  Math Function : Math  Operator=square
  Math Function1 : Math  Operator=square
  Math Function2 : Math  Operator=square
  Sqrt : Sqrt
  Speed : Outport
  wires:
  Longitudinal Velocity/1 -> Math Function1/1
  Lateral Velocity/1 -> Math Function/1
  Sqrt/1 -> Speed/1
  Math Function/1 -> Add/1
  Math Function1/1 -> Add/2
  Add/1 -> Sqrt/1
  Math Function2/1 -> Add/3
  z Velocity/1 -> Math Function2/1

== system TrajectoryFollowVehicleWith14DoF_/Variant Subsystem/StanleyControl_vehicleDynamics/Vehicle Dynamics1/Vehicle Dynamics 14DOF/Delayed Steering System ==
  SteerCmd : Inport
  Add : Sum  Inputs=+-
  Delay : TransferFcn  Denominator=[0.1 0]
  CurrSteer : Outport  VectorParamsAs1DForOutWhenUnconnected=off
  wires:
  Delay/1 -> Add/2, CurrSteer/1
  SteerCmd/1 -> Add/1
  Add/1 -> Delay/1

== system TrajectoryFollowVehicleWith14DoF_/Variant Subsystem/StanleyControl_vehicleDynamics/Vehicle Dynamics1/Vehicle Dynamics 14DOF/Variant Subsystem ==
  note: 1) Add Subsystem or Model blocks as valid variant choices.
      | 2) You cannot connect blocks at this level. At simulation, connectivity is automatically
      | determined, based on the active variant and port name matching.
  VehFdback : Inport
  2DHeightMap : Subsystem  VariantControl="hegihtMap == \"2DMap\""
  CRG : Subsystem  VariantControl="hegihtMap == \"CRG\""
  noElevation : Subsystem  VariantControl="hegihtMap == \"flat\""
  WheelElevation : Outport

== system TrajectoryFollowVehicleWith14DoF_/Variant Subsystem/StanleyControl_vehicleDynamics/Vehicle Dynamics1/Vehicle Dynamics 14DOF/getPoseCG ==
  VehFdbk : Inport
  Bus Selector2 : BusSelector  OutputSignals=Body.InertFrm.Cg.Disp.X,Body.InertFrm.Cg.Disp.Y,Body.InertFrm.Cg.Ang.psi,Body.InertFrm.Cg.Disp.Z,Body.InertFrm.Cg.Ang.theta,Body.InertFrm.Cg.Ang.phi
  Gain{4..7} (4 alike) : Gain  Gain=-1
  Math Function2 : Math  Operator=transpose  SignedPower=on
  Mux2 : Mux  Inputs=6
  Radians to Degrees3 : simulink_extras/Transformations/Radians to Degrees
  Radians to Degrees4 : simulink_extras/Transformations/Radians to Degrees
  Radians to Degrees5 : simulink_extras/Transformations/Radians to Degrees
  pitch : Display  Commented=on
  roll : Display  Commented=on
  x : Display  Commented=on
  y : Display  Commented=on
  yaw : Display  Commented=on
  z : Display  Commented=on
  CurrPose : Outport
  wires:
  Bus Selector2/5 -> Radians to Degrees4/1  "<theta>"
  Bus Selector2/6 -> Radians to Degrees5/1  "<phi>"
  Gain4/1 -> y/1, Mux2/2
  Radians to Degrees5/1 -> roll/1, Mux2/6
  Gain5/1 -> z/1, Mux2/4
  Gain7/1 -> pitch/1, Mux2/5
  Bus Selector2/3 -> Radians to Degrees3/1  "<psi>"
  Bus Selector2/2 -> Gain4/1  "<Y>"
  Bus Selector2/1 -> Mux2/1, x/1  "<X>"
  Gain6/1 -> yaw/1, Mux2/3
  Radians to Degrees4/1 -> Gain7/1
  Mux2/1 -> Math Function2/1
  Bus Selector2/4 -> Gain5/1  "<Z>"
  Radians to Degrees3/1 -> Gain6/1
  Math Function2/1 -> CurrPose/1  "CurrPose"
  VehFdbk/1 -> Bus Selector2/1

== system TrajectoryFollowVehicleWith14DoF_/Variant Subsystem/StanleyControl_vehicleDynamics/Vehicle Dynamics1/Vehicle Dynamics 14DOF/getPoseRear ==
  VehFdbk : Inport
  Bus Selector1 : BusSelector  OutputSignals=Body.InertFrm.RearAxl.Lft.Disp.X,Body.InertFrm.RearAxl.Rght.Disp.X,Body.InertFrm.RearAxl.Lft.Disp.Y,Body.InertFrm.RearAxl.Rght.Disp.Y,Body.InertFrm.Cg.Ang.psi,Body.InertFrm.RearAxl.Lft.Disp.Z,Body.InertFrm.RearAxl.Rght.Disp.Z,Body.InertFrm.Cg.Ang.theta
  Gain{,1..3} (4 alike) : Gain  Gain=-1
  Math Function1 : Math  Operator=transpose  SignedPower=on
  Mean : Subsystem
  Mean1 : Subsystem
  Mean2 : Subsystem
  Mux1 : Mux  Inputs=5
  Radians to Degrees1 : simulink_extras/Transformations/Radians to Degrees
  Radians to Degrees2 : simulink_extras/Transformations/Radians to Degrees
  CurrPose : Outport
  wires:
  Bus Selector1/2 -> Mean/2(<X>1)  "<X>"
  Bus Selector1/1 -> Mean/1(<X>)  "<X>"
  Bus Selector1/5 -> Radians to Degrees1/1  "<psi>"
  Gain1/1 -> Mux1/4
  Bus Selector1/4 -> Mean1/2(<Y>1)  "<Y>"
  Mean1/1(Out1) -> Gain/1
  Gain/1 -> Mux1/2
  Gain3/1 -> Mux1/5
  Bus Selector1/8 -> Radians to Degrees2/1  "<theta>"
  Mean2/1(Out1) -> Gain1/1
  Bus Selector1/3 -> Mean1/1(<Y>)  "<Y>"
  Mean/1(Out1) -> Mux1/1
  Gain2/1 -> Mux1/3
  Radians to Degrees1/1 -> Gain2/1
  Bus Selector1/6 -> Mean2/1(<Z>)  "<Z>"
  Radians to Degrees2/1 -> Gain3/1
  Bus Selector1/7 -> Mean2/2(<Z>1)  "<Z>"
  Mux1/1 -> Math Function1/1
  Math Function1/1 -> CurrPose/1  "CurrPose"
  VehFdbk/1 -> Bus Selector1/1

== system TrajectoryFollowVehicleWith14DoF_/Variant Subsystem/StanleyControl_vehicleDynamics/Vehicle Dynamics1/Vehicle Dynamics 3DOF/Calculate Norm ==
  Lateral Velocity : Inport
  Longitudinal Velocity : Inport  Port=2
  Add : Sum
  Math Function : Math  Operator=square
  Math Function1 : Math  Operator=square
  Sqrt : Sqrt
  Speed : Outport
  wires:
  Add/1 -> Sqrt/1
  Math Function1/1 -> Add/2
  Math Function/1 -> Add/1
  Sqrt/1 -> Speed/1
  Lateral Velocity/1 -> Math Function/1
  Longitudinal Velocity/1 -> Math Function1/1

== system TrajectoryFollowVehicleWith14DoF_/Variant Subsystem/StanleyControl_vehicleDynamics/Vehicle Dynamics1/Vehicle Dynamics 3DOF/Delayed Steering System ==
  SteerCmd : Inport
  Add : Sum  Inputs=+-
  Delay : TransferFcn  Denominator=[0.1 0]
  CurrSteer : Outport  VectorParamsAs1DForOutWhenUnconnected=off
  wires:
  Add/1 -> Delay/1
  SteerCmd/1 -> Add/1
  Delay/1 -> CurrSteer/1, Add/2

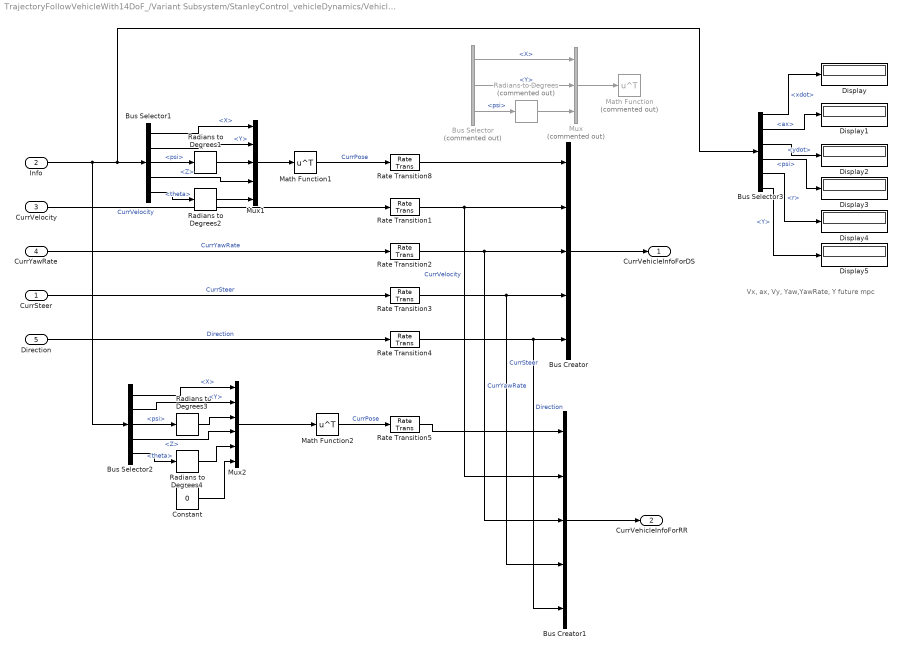
== system TrajectoryFollowVehicleWith14DoF_/Variant Subsystem/StanleyControl_vehicleDynamics/Vehicle Dynamics1/Vehicle Dynamics 3DOF/Pack Current States ==
  note: Vx, ax, Vy, Yaw,YawRate, Y future mpc
  CurrSteer : Inport
  Info : Inport  Port=2
  CurrVelocity : Inport  Port=3
  CurrYawRate : Inport  Port=4
  Direction : Inport  Port=5
  Bus Creator : BusCreator  Inputs=5  OutDataTypeStr=Bus: BusVehicleInfo  NonVirtualBus=on
      settings: InheritFromInputs=off
  Bus Creator1 : BusCreator  Inputs=5  OutDataTypeStr=Bus: BusFullVehicleInfo  NonVirtualBus=on
      settings: InheritFromInputs=off
  Bus Selector : BusSelector  Commented=on  OutputSignals=InertFrm.RearAxl.Disp.X,InertFrm.RearAxl.Disp.Y,InertFrm.Cg.Ang.psi
  Bus Selector1 : BusSelector  OutputSignals=InertFrm.RearAxl.Disp.X,InertFrm.RearAxl.Disp.Y,InertFrm.Cg.Ang.psi,InertFrm.RearAxl.Disp.Z,InertFrm.Cg.Ang.theta
  Bus Selector2 : BusSelector  OutputSignals=InertFrm.Cg.Disp.X,InertFrm.Cg.Disp.Y,InertFrm.Cg.Ang.psi,InertFrm.Cg.Disp.Z,InertFrm.Cg.Ang.theta
  Bus Selector3 : BusSelector  OutputSignals=BdyFrm.Cg.Vel.xdot,BdyFrm.Cg.Acc.ax,BdyFrm.Cg.Vel.ydot,InertFrm.Cg.Ang.psi,BdyFrm.Cg.AngVel.r,InertFrm.Cg.Disp.Y
  Constant : Constant  Value=0
  Display{,1..5} (6 alike) : Display
  Math Function : Math  Commented=on  Operator=transpose  SignedPower=on
  Math Function1 : Math  Operator=transpose  SignedPower=on
  Math Function2 : Math  Operator=transpose  SignedPower=on
  Mux : Mux  Commented=on  Inputs=3
  Mux1 : Mux  Inputs=5
  Mux2 : Mux  Inputs=6
  Radians to Degrees : simulink_extras/Transformations/Radians to Degrees  Commented=on
  Radians to Degrees{1..4} (4 alike) : simulink_extras/Transformations/Radians to Degrees
  Rate Transition{1..5,8} (6 alike) : RateTransition  OutPortSampleTime=timeStep
  CurrVehicleInfoForDS : Outport  VectorParamsAs1DForOutWhenUnconnected=off
  CurrVehicleInfoForRR : Outport  Port=2  VectorParamsAs1DForOutWhenUnconnected=off
  wires:
  CurrVelocity/1 -> Rate Transition1/1  "CurrVelocity"
  CurrSteer/1 -> Rate Transition3/1  "CurrSteer"
  Math Function1/1 -> Rate Transition8/1  "CurrPose"
  CurrYawRate/1 -> Rate Transition2/1  "CurrYawRate"
  Direction/1 -> Rate Transition4/1  "Direction"
  Mux/1 -> Math Function/1
  Radians to Degrees/1 -> Mux/3
  Bus Selector/2 -> Mux/2  "<Y>"
  Bus Selector/1 -> Mux/1  "<X>"
  Bus Selector/3 -> Radians to Degrees/1  "<psi>"
  Bus Creator/1 -> CurrVehicleInfoForDS/1
  Rate Transition8/1 -> Bus Creator/1
  Bus Selector1/4 -> Mux1/4  "<Z>"
  Mux1/1 -> Math Function1/1
  Radians to Degrees1/1 -> Mux1/3
  Bus Selector1/2 -> Mux1/2  "<Y>"
  Bus Selector1/1 -> Mux1/1  "<X>"
  Bus Selector1/5 -> Radians to Degrees2/1  "<theta>"
  Radians to Degrees2/1 -> Mux1/5
  Bus Selector1/3 -> Radians to Degrees1/1  "<psi>"
  Rate Transition1/1 -> Bus Creator1/2, Bus Creator/2  "CurrVelocity"
  Radians to Degrees4/1 -> Mux2/5
  Bus Creator1/1 -> CurrVehicleInfoForRR/1
  Bus Selector2/4 -> Mux2/4  "<Z>"
  Bus Selector2/3 -> Radians to Degrees3/1  "<psi>"
  Rate Transition2/1 -> Bus Creator1/3, Bus Creator/3  "CurrYawRate"
  Radians to Degrees3/1 -> Mux2/3
  Bus Selector2/1 -> Mux2/1  "<X>"
  Rate Transition4/1 -> Bus Creator1/5, Bus Creator/5  "Direction"
  Mux2/1 -> Math Function2/1
  Math Function2/1 -> Rate Transition5/1  "CurrPose"
  Bus Selector2/2 -> Mux2/2  "<Y>"
  Rate Transition3/1 -> Bus Creator1/4, Bus Creator/4  "CurrSteer"
  Info/1 -> Bus Selector2/1, Bus Selector3/1, Bus Selector1/1
  Bus Selector2/5 -> Radians to Degrees4/1  "<theta>"
  Rate Transition5/1 -> Bus Creator1/1
  Constant/1 -> Mux2/6
  Bus Selector3/1 -> Display/1  "<xdot>"
  Bus Selector3/2 -> Display1/1  "<ax>"
  Bus Selector3/3 -> Display2/1  "<ydot>"
  Bus Selector3/4 -> Display3/1  "<psi>"
  Bus Selector3/5 -> Display4/1  "<r>"
  Bus Selector3/6 -> Display5/1  "<Y>"
